simulink model "FixedWingModel"  (R2021a)
settings: configuration reference "ctrlConfigSet" (kept outside this file)
values from neighbouring files (symbols this model uses):
  ap = 0.01    [pathFollowingData.sldd]
  env = 0.0065    [pathFollowingData.sldd]
  sensors = 0.0    [pathFollowingData.sldd]
  uavParam = 2.795    [pathFollowingData.sldd]
undefined symbols (not defined in the file or in its folder): DiscIntNeverNeededParam, Earth, WGS84
libraries: simulink x24, mbdriLib x21, pid_lib x1, simulink_need_slupdate x1, aerolibconvert2 x1, aerolibtransform2 x1, uavalgslib x1
(part 2 of 2)

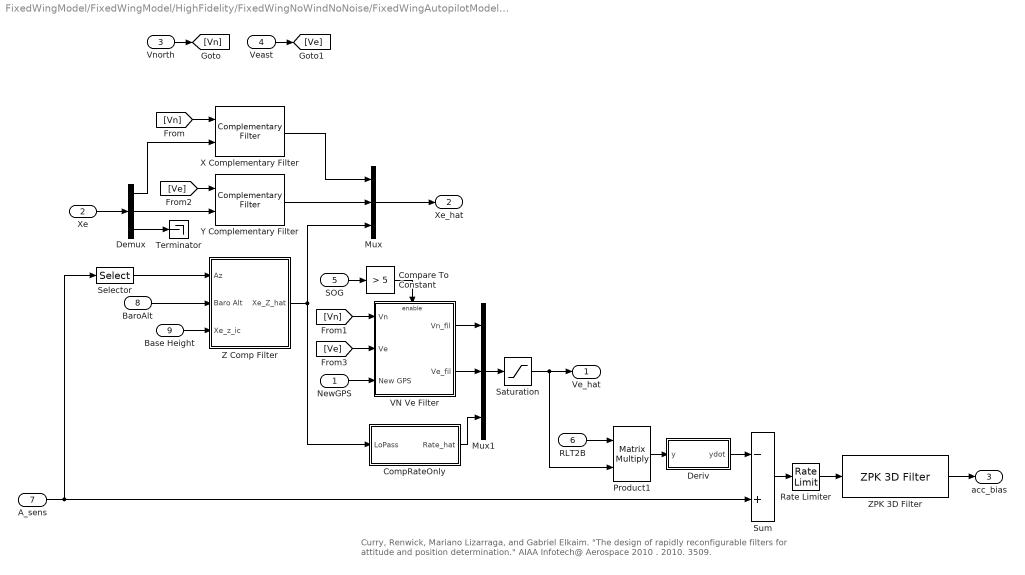
== system FixedWingModel/FixedWingModel/HighFidelity/FixedWingNoWindNoNoise/FixedWingAutopilotModel/Sensor Module/Position Filter/Position&Velocity Filter ==
  note: Curry, Renwick, Mariano Lizarraga, and Gabriel Elkaim. "The design of rapidly reconfigurable filters for attitude and position determination." AIAA Infotech@ Aerospace 2010 . 2010. 3509.
  NewGPS : Inport
  Xe : Inport  Port=2
  Vnorth : Inport  Port=3
  Veast : Inport  Port=4
  SOG : Inport  Port=5
  RLT2B : Inport  Port=6
  A_sens : Inport  Port=7  Unit=m/s^2
  BaroAlt : Inport  Port=8
  Base Height : Inport  Port=9
  CompRateOnly : Subsystem  mask{omega=ap.cf.vzCutoff, T=ap.apSampleTime}
      mask prompts: omega "Cutoff Freq (rad/sec)"; T "Sample Time"
  Compare To Constant : simulink/Logic and Bit Operations/Compare To Constant  relop=>  const=5  OutDataTypeStr=boolean  ZeroCross=off
  Demux : Demux  Outputs=3
  "Deriv " : Subsystem
  Mux : Mux  Inputs=3
  Mux1 : Mux  Inputs=3
  Product1 : Product  Multiplication=Matrix(*)  RndMeth=Zero
  Rate Limiter : RateLimiter  RisingSlewLimit=ap.cf.accBiasRateLimit  FallingSlewLimit=-ap.cf.accBiasRateLimit  SampleTimeMode=inherited
  Saturation : Saturate  UpperLimit=40  LowerLimit=-40
      settings: AttributesFormatString="[%<LowerLimit>  %<UpperLimit>]"
  Selector : Selector  InputPortWidth=3  IndexOptions=Index vector (dialog)  Indices=[3]  OutputSizes=1
  Sum : Sum  Inputs=-+  OutDataTypeStr=single
  Terminator : Terminator
  VN Ve Filter : Subsystem
  X Complementary Filter : mbdriLib/Filtering/Complementary Filter  omega=ap.cf.xCutoff  T=ap.apSampleTime
  Y Complementary Filter : mbdriLib/Filtering/Complementary Filter  omega=ap.cf.yCutoff  T=ap.apSampleTime
  Z Comp Filter : Subsystem
  ZPK 3D Filter : mbdriLib/Filtering/ZPK 3D Filter  zval=[]  pval=-1/ap.cf.accBiasRateLimit  kval=1  TSample=ap.apSampleTime
  Ve_hat : Outport  VectorParamsAs1DForOutWhenUnconnected=off
  Xe_hat : Outport  Port=2  VectorParamsAs1DForOutWhenUnconnected=off
  acc_bias : Outport  Port=3  Unit=m/s^2  VectorParamsAs1DForOutWhenUnconnected=off
  wires:
  Saturation/1 -> Ve_hat/1, Product1/2
  Z Comp Filter/1(Xe_Z_hat) -> Mux/3, CompRateOnly/1(LoPass)
  BaroAlt/1 -> Z Comp Filter/2(Baro Alt)
  Demux/3 -> Terminator/1
  Selector/1 -> Z Comp Filter/1(Az)
  [Ve] -> VN Ve Filter/2(Ve)
  [Ve] -> Y Complementary Filter/1
  Veast/1 -> [Ve]
  [Vn] -> VN Ve Filter/1(Vn)
  [Vn] -> X Complementary Filter/1
  Vnorth/1 -> [Vn]
  CompRateOnly/1(Rate_hat) -> Mux1/3
  VN Ve Filter/2(Ve_fil) -> Mux1/2
  VN Ve Filter/1(Vn_fil) -> Mux1/1
  Mux/1 -> Xe_hat/1
  X Complementary Filter/1 -> Mux/1
  Y Complementary Filter/1 -> Mux/2
  Demux/2 -> Y Complementary Filter/2
  Demux/1 -> X Complementary Filter/2
  Xe/1 -> Demux/1
  Mux1/1 -> Saturation/1
  NewGPS/1 -> VN Ve Filter/3(New GPS)
  Compare To Constant/1 -> VN Ve Filter/Enable
  SOG/1 -> Compare To Constant/1
  Rate Limiter/1 -> ZPK 3D Filter/1
  ZPK 3D Filter/1 -> acc_bias/1
  Sum/1 -> Rate Limiter/1
  Product1/1 -> "Deriv "/1(y)
  "Deriv "/1(ydot) -> Sum/1
  A_sens/1 -> Selector/1, Sum/2
  RLT2B/1 -> Product1/1
  Base Height/1 -> Z Comp Filter/3(Xe_z_ic)

== system FixedWingModel/FixedWingModel/HighFidelity/FixedWingNoWindNoNoise/FixedWingAutopilotModel/InnerLoopAutopilot/Longitudinal Channel/Rate Limiter Dynamic with External IC and Autoreset for Change in IC/Subsystem ==
  WP Fly : Inport
  Compare To Constant : simulink/Logic and Bit Operations/Compare To Constant  relop=>=  const=0.5  OutDataTypeStr=boolean
  Compare To Constant1 : simulink/Logic and Bit Operations/Compare To Constant  relop=<  const=0.5  OutDataTypeStr=boolean
  Logical Operator : Logic  AllPortsSameDT=off  OutDataTypeStr=boolean
  Unit Delay : UnitDelay  SampleTime=-1  HasFrameUpgradeWarning=on
  Just Enab : Outport  VectorParamsAs1DForOutWhenUnconnected=off
  wires:
  WP Fly/1 -> Unit Delay/1, Compare To Constant/1
  Compare To Constant/1 -> Logical Operator/1
  Compare To Constant1/1 -> Logical Operator/2
  Unit Delay/1 -> Compare To Constant1/1
  Logical Operator/1 -> Just Enab/1

== system FixedWingModel/FixedWingModel/HighFidelity/FixedWingNoWindNoNoise/FixedWingAutopilotModel/Sensor Module/Position Filter/Get Vn Ve/Subsystem5 ==
  u : Inport
  Trigonometric Function : Trigonometry
  Trigonometric Function1 : Trigonometry  Operator=cos
  sin(u) : Outport  VectorParamsAs1DForOutWhenUnconnected=off
  cos(u) : Outport  Port=2  VectorParamsAs1DForOutWhenUnconnected=off
  wires:
  u/1 -> Trigonometric Function/1, Trigonometric Function1/1
  Trigonometric Function/1 -> sin(u)/1
  Trigonometric Function1/1 -> cos(u)/1

== system FixedWingModel/FixedWingModel/HighFidelity/FixedWingNoWindNoNoise/FixedWingAutopilotModel/Sensor Module/Position Filter/Position&Velocity Filter/CompRateOnly ==
  LoPass : Inport
  Gain : Gain  Gain=omega
      settings: AttributesFormatString=%<Gain>
  Sum1 : Sum  Inputs=|+-
  Unit Delay : UnitDelay  SampleTime=T  HasFrameUpgradeWarning=on
  ZPK 1D Discrete Filter : mbdriLib/Filtering/ZPK 1D Discrete Filter  zval=[]  pval=[0]  kval=1  TSample=0.01
  Rate_hat : Outport  VectorParamsAs1DForOutWhenUnconnected=off
  wires:
  Unit Delay/1 -> Sum1/2
  LoPass/1 -> Sum1/1
  Sum1/1 -> Gain/1
  Gain/1 -> ZPK 1D Discrete Filter/1, Rate_hat/1
  ZPK 1D Discrete Filter/1 -> Unit Delay/1

== system FixedWingModel/FixedWingModel/HighFidelity/FixedWingNoWindNoNoise/FixedWingAutopilotModel/Sensor Module/Position Filter/Position&Velocity Filter/Deriv  ==
  y : Inport
  Gain2 : Gain  Gain=[ 1/(5*ap.apSampleTime) ]
      settings: AttributesFormatString=%<Gain>
  Integer Delay1 : Delay  DelayLength=5  InitialCondition=0  SampleTime=ap.apSampleTime
  Sum5 : Sum  Inputs=-+|
  ydot : Outport  VectorParamsAs1DForOutWhenUnconnected=off
  wires:
  Gain2/1 -> ydot/1
  y/1 -> Integer Delay1/1, Sum5/2
  Integer Delay1/1 -> Sum5/1
  Sum5/1 -> Gain2/1

== system FixedWingModel/FixedWingModel/HighFidelity/FixedWingNoWindNoNoise/FixedWingAutopilotModel/Sensor Module/Position Filter/Position&Velocity Filter/VN Ve Filter ==
  Vn : Inport
  Ve : Inport  Port=2
  New GPS : Inport  Port=3
  Enable : EnablePort
  Constant : Constant  Value=ap.apSampleTime
      settings: AttributesFormatString=%<Value>
  RateAid for GPS : mbdriLib/Filtering/RateAid for GPS  SystemSampleTime=-1  VariantActivationTime=update diagram  Latency=0  AutoFrameSizeCalculation=off
  RateAid for GPS1 : mbdriLib/Filtering/RateAid for GPS  SystemSampleTime=-1  VariantActivationTime=update diagram  Latency=0  AutoFrameSizeCalculation=off
  Vn_fil : Outport  OutputWhenDisabled=reset  InitialOutput=0  VectorParamsAs1DForOutWhenUnconnected=off
  Ve_fil : Outport  Port=2  OutputWhenDisabled=reset  InitialOutput=0  VectorParamsAs1DForOutWhenUnconnected=off
  wires:
  Constant/1 -> RateAid for GPS1/3, RateAid for GPS/3
  New GPS/1 -> RateAid for GPS/2, RateAid for GPS1/2
  Vn/1 -> RateAid for GPS/1
  Ve/1 -> RateAid for GPS1/1
  RateAid for GPS/1 -> Vn_fil/1
  RateAid for GPS1/1 -> Ve_fil/1

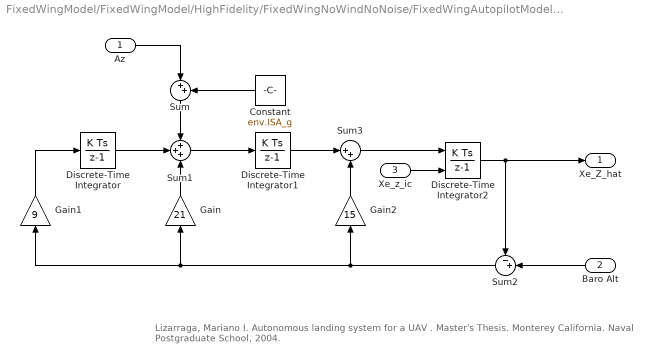
== system FixedWingModel/FixedWingModel/HighFidelity/FixedWingNoWindNoNoise/FixedWingAutopilotModel/Sensor Module/Position Filter/Position&Velocity Filter/Z Comp Filter ==
  note: Lizarraga, Mariano I. Autonomous landing system for a UAV . Master's Thesis. Monterey California. Naval Postgraduate School, 2004.
  Az : Inport
  Baro Alt : Inport  Port=2
  Xe_z_ic : Inport  Port=3
  Constant : Constant  Value=env.ISA_g  OutDataTypeStr=single
      settings: AttributesFormatString=%<Value>
  Discrete-Time Integrator : DiscreteIntegrator  gainval=1  SampleTime=-1  ICPrevOutput=DiscIntNeverNeededParam  ICPrevScaledInput=DiscIntNeverNeededParam
  Discrete-Time Integrator1 : DiscreteIntegrator  gainval=1  SampleTime=-1  ICPrevOutput=DiscIntNeverNeededParam  ICPrevScaledInput=DiscIntNeverNeededParam
  Discrete-Time Integrator2 : DiscreteIntegrator  gainval=1  InitialConditionSource=external  SampleTime=-1  ICPrevOutput=DiscIntNeverNeededParam  ICPrevScaledInput=DiscIntNeverNeededParam
  Gain : Gain  Gain=21  OutDataTypeStr=single
      settings: AttributesFormatString=%<Gain>
  Gain1 : Gain  Gain=9  OutDataTypeStr=single
      settings: AttributesFormatString=%<Gain>
  Gain2 : Gain  Gain=15  OutDataTypeStr=single
      settings: AttributesFormatString=%<Gain>
  Sum : Sum  Inputs=|++
  Sum1 : Sum  Inputs=+++
  Sum2 : Sum  Inputs=-+|
  Sum3 : Sum  Inputs=|++
  Xe_Z_hat : Outport  VectorParamsAs1DForOutWhenUnconnected=off
  wires:
  Discrete-Time Integrator2/1 -> Sum2/1, Xe_Z_hat/1
  Gain2/1 -> Sum3/2
  Gain1/1 -> Discrete-Time Integrator/1
  Gain/1 -> Sum1/3
  Sum2/1 -> Gain2/1, Gain/1, Gain1/1
  Sum3/1 -> Discrete-Time Integrator2/1
  Discrete-Time Integrator1/1 -> Sum3/1
  Baro Alt/1 -> Sum2/2
  Xe_z_ic/1 -> Discrete-Time Integrator2/2
  Sum1/1 -> Discrete-Time Integrator1/1
  Sum/1 -> Sum1/1
  Discrete-Time Integrator/1 -> Sum1/2
  Constant/1 -> Sum/2
  Az/1 -> Sum/1
